simulink model "adip_gs_servo_sim"  (R2013a)
settings: Solver=ode4  SolverMode=SingleTasking  StartTime=0.0  StopTime=12  FixedStep=0.001  RelTol=1e-3
values from neighbouring files (symbols this model uses):
  a1 = vertex(1,i)    [p2c13_ex5_adip_lqr_servo.m]    (also in p2c13_ex5_adip_oc_nominal_servo.m; p2c13_ex5_adip_oc_robust_servo.m)
  b1 = vertex(2,i)    [p2c13_ex5_adip_lqr_servo.m]    (also in p2c13_ex5_adip_oc_nominal_servo.m; p2c13_ex5_adip_oc_robust_servo.m)
  d0 = 0    [p2c122_ex4_adip_oc_multiobjective_servo.m]    (also in p2c122_ex4_adip_oc_servo.m; p2c13_ex5_adip_lqr_servo.m; p2c13_ex5_adip_oc_nominal_servo.m; p2c13_ex5_adip_oc_robust_servo.m)
  dtheta1_0 = 0    [p2c122_ex4_adip_oc_multiobjective_servo.m]    (also in p2c122_ex4_adip_oc_servo.m; p2c13_ex5_adip_lqr_servo.m; p2c13_ex5_adip_oc_nominal_servo.m; p2c13_ex5_adip_oc_robust_servo.m)
  dtheta2_0 = 0    [p2c122_ex4_adip_oc_multiobjective_servo.m]    (also in p2c122_ex4_adip_oc_servo.m; p2c13_ex5_adip_lqr_servo.m; p2c13_ex5_adip_oc_nominal_servo.m; p2c13_ex5_adip_oc_robust_servo.m)
  L_0 = double(L_0)    [p2c15_ex7_adip_oc_gs_servo.m]    (also in p2c15_ex7_adip_oc_gs_servo_old.m)
  L_1 = double(L_1)    [p2c15_ex7_adip_oc_gs_servo.m]    (also in p2c15_ex7_adip_oc_gs_servo_old.m)
  L_2 = double(L_2)    [p2c15_ex7_adip_oc_gs_servo.m]    (also in p2c15_ex7_adip_oc_gs_servo_old.m)
  r0 = 30*pi/180    (= 0.523598775598)    [p2c122_ex4_adip_oc_multiobjective_servo.m]    (also in p2c122_ex4_adip_oc_servo.m; p2c13_ex5_adip_lqr_servo.m; p2c13_ex5_adip_oc_nominal_servo.m; p2c13_ex5_adip_oc_robust_servo.m)
  t_dis = 0    [p2c122_ex4_adip_oc_multiobjective_servo.m]    (also in p2c122_ex4_adip_oc_servo.m; p2c13_ex5_adip_lqr_servo.m; p2c13_ex5_adip_oc_nominal_servo.m; p2c13_ex5_adip_oc_robust_servo.m)
  theta1_0 = 0    [p2c122_ex4_adip_oc_multiobjective_servo.m]    (also in p2c122_ex4_adip_oc_servo.m; p2c13_ex5_adip_lqr_servo.m; p2c13_ex5_adip_oc_nominal_servo.m; p2c13_ex5_adip_oc_robust_servo.m)
  theta2_0 = 0    [p2c122_ex4_adip_oc_multiobjective_servo.m]    (also in p2c122_ex4_adip_oc_servo.m; p2c13_ex5_adip_lqr_servo.m; p2c13_ex5_adip_oc_nominal_servo.m; p2c13_ex5_adip_oc_robust_servo.m)
  X_0 = double(X_0)    [p2c15_ex7_adip_oc_gs_servo.m]    (also in p2c15_ex7_adip_oc_gs_servo_old.m)
  X_1 = double(X_1)    [p2c15_ex7_adip_oc_gs_servo.m]    (also in p2c15_ex7_adip_oc_gs_servo_old.m)
  X_2 = double(X_2)    [p2c15_ex7_adip_oc_gs_servo.m]    (also in p2c15_ex7_adip_oc_gs_servo_old.m)
undefined symbols (not defined in the file or in its folder): alpha2, alpha3, alpha5, mu2
settings Model: Creator=kawata  LastModifiedBy=kawata
settings DataIOCC: SignalLoggingSaveFormat=ModelDataLogs
settings OptimizationCC: BlockReduction=off  BooleanDataType=off
settings DebuggingCC: SaveWithParameterizedLinksMsg=none  SignalResolutionControl=TryResolveAllWithWarning  SolverPrmCheckMsg=none  MultiTaskDSMMsg=warning  MultiTaskCondExecSysMsg=none  StrictBusMsg=None
settings HardwareCC: TargetUnknown=on
settings RTWCC: IncludeERTFirstTime=on

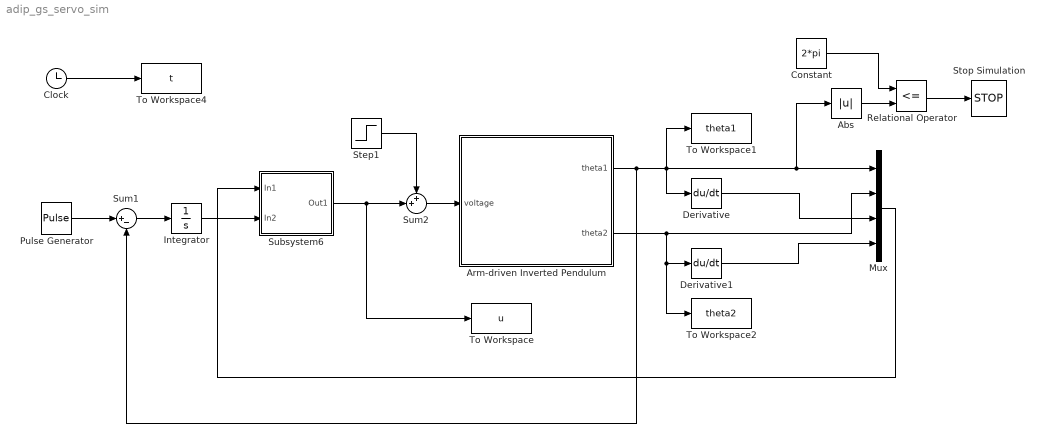
== system adip_gs_servo_sim ==
  Abs : Abs
  Arm-driven Inverted Pendulum : Subsystem
      mask Display: image(imread('adip.jpg'),'center')
  Clock : Clock
  Constant : Constant  Value=2*pi
  Derivative : Derivative
  Derivative1 : Derivative
  Integrator : Integrator
  Mux : Mux
  Pulse Generator : DiscretePulseGenerator  PulseType=Time based  Amplitude=r0  Period=12  PulseWidth=50
  Relational Operator : RelationalOperator  Operator=<=  OutDataTypeStr=boolean
  Step1 : Step  Time=t_dis  After=d0  SampleTime=0
  Stop Simulation : Stop
  Subsystem6 : Subsystem
  Sum1 : Sum  Inputs=|+-  SaturateOnIntegerOverflow=on  InputSameDT=on  OutDataTypeStr=Inherit: Same as first input
  Sum2 : Sum  Inputs=++|  SaturateOnIntegerOverflow=on  InputSameDT=on  OutDataTypeStr=Inherit: Same as first input
  To Workspace : ToWorkspace  VariableName=u  SampleTime=-1
  To Workspace1 : ToWorkspace  VariableName=theta1  SampleTime=-1
  To Workspace2 : ToWorkspace  VariableName=theta2  SampleTime=-1
  To Workspace4 : ToWorkspace  VariableName=t  SampleTime=-1
  wires:
  Sum1/1 -> Integrator/1
  Subsystem6/1(Out1) -> Sum2/2, To Workspace/1
  Pulse Generator/1 -> Sum1/1
  Step1/1 -> Sum2/1
  Sum2/1 -> Arm-driven Inverted Pendulum/1(voltage)
  Clock/1 -> To Workspace4/1
  Arm-driven Inverted Pendulum/1(theta1) -> To Workspace1/1, Derivative/1, Abs/1, Mux/1, Sum1/2
  Arm-driven Inverted Pendulum/2(theta2) -> To Workspace2/1, Derivative1/1, Mux/2
  Derivative/1 -> Mux/3
  Derivative1/1 -> Mux/4
  Mux/1 -> Subsystem6/1(In1)
  Integrator/1 -> Subsystem6/2(In2)
  Constant/1 -> Relational Operator/1
  Abs/1 -> Relational Operator/2
  Relational Operator/1 -> Stop Simulation/1

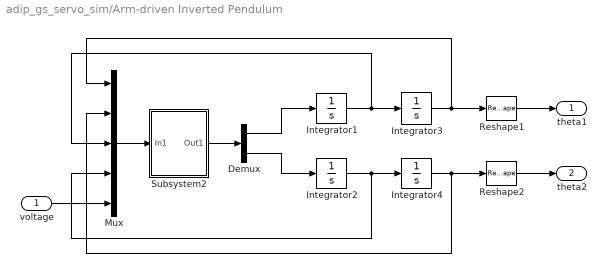
== system adip_gs_servo_sim/Arm-driven Inverted Pendulum ==
  voltage : Inport
  Demux : Demux  Outputs=2
  Integrator1 : Integrator  InitialCondition=dtheta1_0
  Integrator2 : Integrator  InitialCondition=dtheta2_0
  Integrator3 : Integrator  InitialCondition=theta1_0
  Integrator4 : Integrator  InitialCondition=theta2_0
  Mux : Mux  Inputs=5
  Reshape1 : Reshape
  Reshape2 : Reshape
  Subsystem2 : Subsystem
  theta1 : Outport
  theta2 : Outport  Port=2
  wires:
  voltage/1 -> Mux/5
  Integrator4/1 -> Mux/2, Reshape2/1
  Integrator3/1 -> Mux/1, Reshape1/1
  Integrator2/1 -> Integrator4/1, Mux/4
  Integrator1/1 -> Integrator3/1, Mux/3
  Demux/2 -> Integrator2/1
  Demux/1 -> Integrator1/1
  Mux/1 -> Subsystem2/1(In1)
  Subsystem2/1(Out1) -> Demux/1
  Reshape2/1 -> theta2/1
  Reshape1/1 -> theta1/1

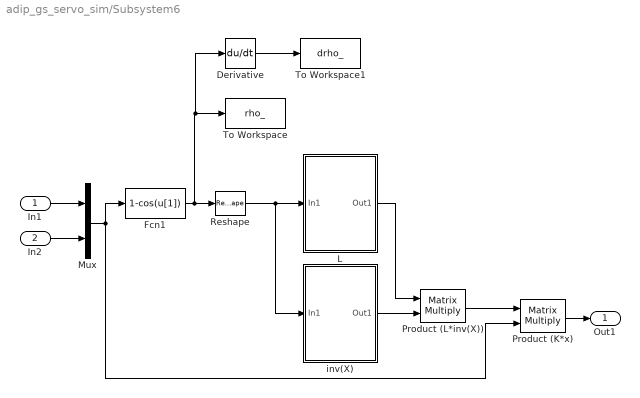
== system adip_gs_servo_sim/Subsystem6 ==
  In1 : Inport
  In2 : Inport  Port=2
  Derivative : Derivative
  Fcn1 : Fcn  Expr=1-cos(u[1])
  L : Subsystem
  Mux : Mux  Inputs=2
  Product (K*x) : Product  Multiplication=Matrix(*)  SaturateOnIntegerOverflow=on  InputSameDT=on  OutDataTypeStr=Inherit: Same as first input
  Product (L*inv(X)) : Product  Multiplication=Matrix(*)  SaturateOnIntegerOverflow=on  InputSameDT=on  OutDataTypeStr=Inherit: Same as first input
  Reshape : Reshape
  To Workspace : ToWorkspace  VariableName=rho_  SampleTime=-1
  To Workspace1 : ToWorkspace  VariableName=drho_  SampleTime=-1
  inv(X) : Subsystem
  Out1 : Outport
  wires:
  Product (K*x)/1 -> Out1/1
  Mux/1 -> Fcn1/1, Product (K*x)/2
  In2/1 -> Mux/2
  In1/1 -> Mux/1
  Fcn1/1 -> Derivative/1, To Workspace/1, Reshape/1
  inv(X)/1(Out1) -> Product (L*inv(X))/2
  L/1(Out1) -> Product (L*inv(X))/1
  Product (L*inv(X))/1 -> Product (K*x)/1
  Reshape/1 -> inv(X)/1(In1), L/1(In1)
  Derivative/1 -> To Workspace1/1

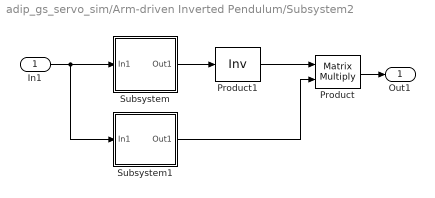
== system adip_gs_servo_sim/Arm-driven Inverted Pendulum/Subsystem2 ==
  In1 : Inport
  Product : Product  Multiplication=Matrix(*)  SaturateOnIntegerOverflow=on  InputSameDT=on  OutDataTypeStr=Inherit: Same as first input
  Product1 : Product  Inputs=/  Multiplication=Matrix(*)  SaturateOnIntegerOverflow=on  InputSameDT=on  OutDataTypeStr=Inherit: Same as first input
  Subsystem : Subsystem
  Subsystem1 : Subsystem
  Out1 : Outport
  wires:
  Subsystem/1(Out1) -> Product1/1
  Product1/1 -> Product/1
  Subsystem1/1(Out1) -> Product/2
  In1/1 -> Subsystem/1(In1), Subsystem1/1(In1)
  Product/1 -> Out1/1

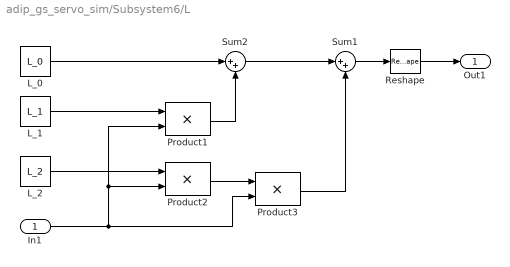
== system adip_gs_servo_sim/Subsystem6/L ==
  In1 : Inport
  L_0 : Constant  Value=L_0
  L_1 : Constant  Value=L_1
  L_2 : Constant  Value=L_2
  Product1 : Product  SaturateOnIntegerOverflow=on  InputSameDT=on  OutDataTypeStr=Inherit: Same as first input
  Product2 : Product  SaturateOnIntegerOverflow=on  InputSameDT=on  OutDataTypeStr=Inherit: Same as first input
  Product3 : Product  SaturateOnIntegerOverflow=on  InputSameDT=on  OutDataTypeStr=Inherit: Same as first input
  Reshape : Reshape  OutputDimensionality=Row vector (2-D)
  Sum1 : Sum  Inputs=|++  SaturateOnIntegerOverflow=on  InputSameDT=on  OutDataTypeStr=Inherit: Same as first input
  Sum2 : Sum  Inputs=|++  SaturateOnIntegerOverflow=on  InputSameDT=on  OutDataTypeStr=Inherit: Same as first input
  Out1 : Outport
  wires:
  L_0/1 -> Sum2/1
  L_1/1 -> Product1/1
  Product1/1 -> Sum2/2
  Reshape/1 -> Out1/1
  In1/1 -> Product3/2, Product1/2, Product2/2
  Sum2/1 -> Sum1/1
  Sum1/1 -> Reshape/1
  L_2/1 -> Product2/1
  Product2/1 -> Product3/1
  Product3/1 -> Sum1/2

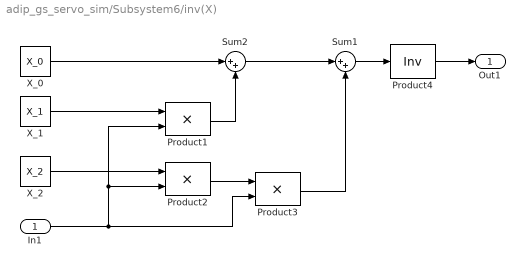
== system adip_gs_servo_sim/Subsystem6/inv(X) ==
  In1 : Inport
  Product1 : Product  SaturateOnIntegerOverflow=on  InputSameDT=on  OutDataTypeStr=Inherit: Same as first input
  Product2 : Product  SaturateOnIntegerOverflow=on  InputSameDT=on  OutDataTypeStr=Inherit: Same as first input
  Product3 : Product  SaturateOnIntegerOverflow=on  InputSameDT=on  OutDataTypeStr=Inherit: Same as first input
  Product4 : Product  Inputs=/  Multiplication=Matrix(*)  SaturateOnIntegerOverflow=on  InputSameDT=on  OutDataTypeStr=Inherit: Same as first input
  Sum1 : Sum  Inputs=|++  SaturateOnIntegerOverflow=on  InputSameDT=on  OutDataTypeStr=Inherit: Same as first input
  Sum2 : Sum  Inputs=|++  SaturateOnIntegerOverflow=on  InputSameDT=on  OutDataTypeStr=Inherit: Same as first input
  X_0 : Constant  Value=X_0
  X_1 : Constant  Value=X_1
  X_2 : Constant  Value=X_2
  Out1 : Outport
  wires:
  Product4/1 -> Out1/1
  X_0/1 -> Sum2/1
  X_1/1 -> Product1/1
  Product1/1 -> Sum2/2
  In1/1 -> Product3/2, Product1/2, Product2/2
  Sum2/1 -> Sum1/1
  Sum1/1 -> Product4/1
  X_2/1 -> Product2/1
  Product2/1 -> Product3/1
  Product3/1 -> Sum1/2

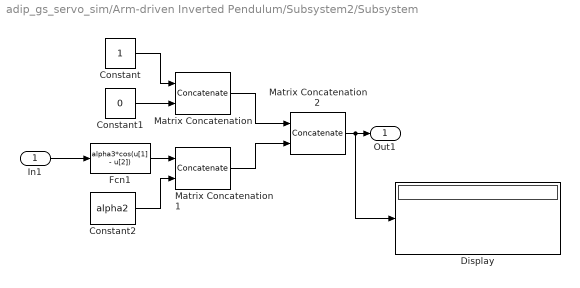
== system adip_gs_servo_sim/Arm-driven Inverted Pendulum/Subsystem2/Subsystem ==
  In1 : Inport
  Constant : Constant
  Constant1 : Constant  Value=0
  Constant2 : Constant  Value=alpha2
  Display : Display
  Fcn1 : Fcn  Expr=alpha3*cos(u[1] - u[2])
  Matrix Concatenation : Concatenate  Mode=Multidimensional array  ConcatenateDimension=2
  Matrix Concatenation1 : Concatenate  Mode=Multidimensional array  ConcatenateDimension=2
  Matrix Concatenation2 : Concatenate  Mode=Multidimensional array
  Out1 : Outport
  wires:
  Constant2/1 -> Matrix Concatenation1/2
  Fcn1/1 -> Matrix Concatenation1/1
  In1/1 -> Fcn1/1
  Matrix Concatenation/1 -> Matrix Concatenation2/1
  Matrix Concatenation1/1 -> Matrix Concatenation2/2
  Matrix Concatenation2/1 -> Display/1, Out1/1
  Constant/1 -> Matrix Concatenation/1
  Constant1/1 -> Matrix Concatenation/2

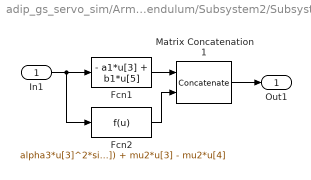
== system adip_gs_servo_sim/Arm-driven Inverted Pendulum/Subsystem2/Subsystem1 ==
  In1 : Inport
  Fcn1 : Fcn  Expr=- a1*u[3] + b1*u[5]
  Fcn2 : Fcn  Expr=alpha3*u[3]^2*sin(u[1] - u[2]) + alpha5*sin(u[2]) + mu2*u[3] - mu2*u[4]
  Matrix Concatenation1 : Concatenate  Mode=Multidimensional array
  Out1 : Outport
  wires:
  Fcn2/1 -> Matrix Concatenation1/2
  Fcn1/1 -> Matrix Concatenation1/1
  In1/1 -> Fcn2/1, Fcn1/1
  Matrix Concatenation1/1 -> Out1/1
